simulink model "yamashev"  (R2015a)
settings: Solver=ode3  StartTime=0.0  StopTime=60.0  RelTol=1e-3
libraries: simulink x2, arduinolib x1
settings Model: ExtModeTrigDuration=2  Creator=maxim  LastModifiedBy=maxim
settings OptimizationCC: OptimizeModelRefInitCode=on  LifeSpan=1
settings DebuggingCC: UnderspecifiedInitializationDetection=Classic  MergeDetectMultiDrivingBlocksExec=none
settings HardwareCC: ProdBitPerInt=16  ProdBitPerPointer=8  ProdIntDivRoundTo=Zero  ProdEndianess=LittleEndian  ProdWordSize=8  ProdHWDeviceType=Atmel->AVR
settings RTWCC: SystemTargetFile=realtime.tlc  GenerateMakefile=off  TemplateMakefile=realtime.tmf  Description=Run on Target Hardware  RTWVerbose=off  CustomInclude=C:\Users\maxim\Documents\Arduino\libraries\OneWire C:\MATLAB\SupportPackages\R2015a\arduino-1.0.5\libraries\LiquidCrystal  CustomSource=C:\Users\maxim\Documents\Arduino\libraries\OneWire\OneWire.cpp C:\MATLAB\SupportPackages\R2015a\arduino-1.0.5\libraries\LiquidCrystal\LiquidCrystal.cpp DS18B20_03_custom.cpp LCD1602_02_custom.cpp
settings ERTTargetCC: CombineOutputUpdateFcns=off  ExtModeTransport=3  ExtModeMexFile=ext_serial_win32_comm_rtt  ExtModeMexArgs=0 1 9600  ERTSrcFileBannerTemplate=realtime_code_template.cgt  ERTHdrFileBannerTemplate=realtime_code_template.cgt  ERTDataSrcFileTemplate=realtime_code_template.cgt  ERTDataHdrFileTemplate=realtime_code_template.cgt  ERTCustomFileTemplate=realtime_file_process.tlc

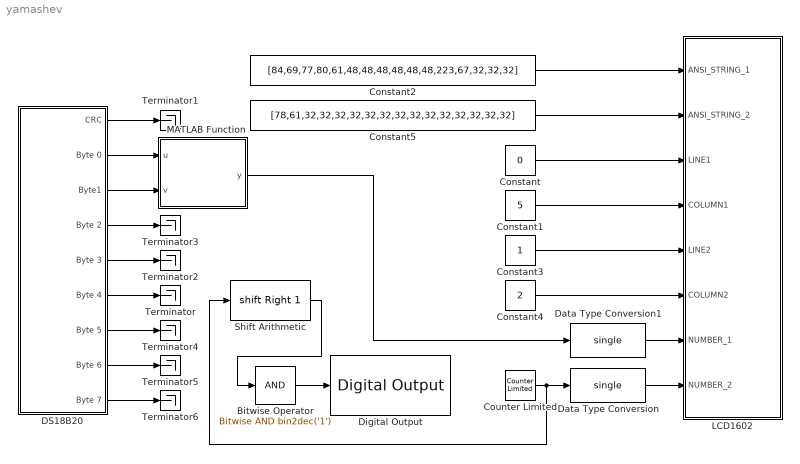
== system yamashev ==
  Bitwise Operator : simulink/Logic and Bit Operations/Bitwise Operator  logicop=AND  UseBitMask=on  BitMask=bin2dec('1')  BitMaskRealWorld=Stored Integer
  Constant : Constant  Value=0  OutDataTypeStr=uint8  LockScale=on
  Constant1 : Constant  Value=5  OutDataTypeStr=uint8  LockScale=on
  Constant2 : Constant  Value=[84,69,77,80,61,48,48,48,48,48,48,223,67,32,32,32]  OutDataTypeStr=fixdt('uint8', 'DataTypeOverride', 'Off')
  Constant3 : Constant  OutDataTypeStr=uint8
  Constant4 : Constant  Value=2  OutDataTypeStr=uint8  LockScale=on
  Constant5 : Constant  Value=[78,61,32,32,32,32,32,32,32,32,32,32,32,32,32,32]  OutDataTypeStr=uint8
  Counter Limited : simulink/Sources/Counter Limited  uplimit=100000  tsamp=-1
  DS18B20 : Subsystem  mask(DS18B20){PIN=34}
      mask prompts: PIN "PIN NUMBER"
      mask help:
      | Блок DS18B20 выполняет функции инициализации и считывания
      | измерений от цифрового термометра DS18B20, подключенного
      | по шине 1-Wire к отладочной плате Arduino Uno.
      | Параметры:
      | Pin Number: номер вывода отладочной платы Arduino Uno для
      | связи с DS18B20.
      | Выходные переменные:
      | CRC:8-разрядное значение контрольной суммы получаемое
      | от цифрового термометра DS18B20.
      | Byte0 ... Byte 7: байты пакета данных, передаваемые
      | от DS18B20.
      | Byte0: LSB младший 8-разрядный регистр температуры.
      | Byte1: MSB старший 8-разрядный регистр температуры.
      mask Help:
      | Блок DS18B20 выполняет функции инициализации и считывания измерений от
      | цифрового термометра DS18B20, подключенного по шине 1-Wire к порту
      | Pin Number отладочной платы Arduino Uno.
      | Параметры:
      | Pin Number: номер вывода Arduino Uno для связи с DS18B20.
      | Выходные переменные:
      | CRC: значение контрольной суммы получаемое от цифрового термометра DS18B20.
      | Byte0 ... Byte 7: байты пакета данных, передаваемые от DS18B20.
      | Byte0: LSB младший 8-разрядный регистр температуры.
      | Byte1: MSB старший 8-разрядный регистр температуры.
  Data Type Conversion : DataTypeConversion  OutDataTypeStr=single
  Data Type Conversion1 : DataTypeConversion  OutDataTypeStr=single
  Digital Output : arduinolib/Digital Output  pinNumber=32  blockPlatform=arduino
  LCD1602 : Subsystem  mask(LCD1602){RS=8, EN=9, D4=4, D5=5, D6=6, D7=7, CURSOR=0}
      mask prompts: RS "RS PIN"; EN "EN PIN"; D4 "D4 PIN"; D5 "D5 PIN"; D6 "D6 PIN"; D7 "D7 PIN"; CURSOR "CURSOR 1-ON 0-OFF"
      mask help:
      | Блок LCD1602 выполняет функции инициализации и вывода
      | информации на двухстрочный 16-символьный алфавитно-цифровой
      | ЖКИ-дисплей.Блок предназначен для работы на микроконтроллере
      | ATmega328 отладочной платы Arduino Uno в 4-битном режиме.
      | Параметры блока:
      | RS номер вывода Arduino Uno, подключаемый к контакту RS ЖКИ.
      | EN номер вывода Arduino Uno, подключаемый к контакту EN ЖКИ.
      | D4 номер вывода Arduino Uno, подключаемый к контакту D4 ЖКИ.
      | D5 номер вывода Arduino Uno, подключаемый к контакту D5 ЖКИ.
      | D6 номер вывода Arduino Uno, подключаемый к контакту D6 ЖКИ.
      | D7 номер вывода Arduino Uno, подключаемый к контакту D7 ЖКИ.
      | CURSOR: 1 – отображение курсора включено;
      |         0 – отображение курсора включено.
      | Входные переменные:
      | ANSI_STRING_1: 16-разрядный массив ANSI-кодов символов для вывода
      | на первую строку ЖКИ. (см. таблицу кодировок дисплея)
      | ANSI_STRING_1: 16-разрядный массив ANSI-кодов символов для вывода
      | на вторую строку ЖКИ. (см. таблицу кодировок дисплея)
      | LINE_1: 0/1 – номер строки для установки курсора вывода числа NUMBER_1.
      | COLUMN_1: 0, 1…15 – номер знакоместе в строке для установки курсора
      | вывода числа NUMBER_1.
      | LINE_2: 0/1 – номер строки для установки курсора вывода числа NUMBER_2.
      | COLUMN_2: 0, 1…15 – номер знакоместе в строке для установки курсора
      | вывода числа NUMBER_2.
      | NUMBER_1: первое числовое значение для отображения на дисплее.
      | NUMBER_2: второе числовое значение для отображения на дисплее.
      mask Help:
      | Блок LCD1602 выполняет функции инициализации и вывода информации на
      | двухстрочный 16-символьный алфавитно-цифровой ЖКИ-дисплей.
      | Блок предназначен для работы на микроконтроллере ATmega328 отладочной платы
      | Arduino Uno только в 4-битном режиме.
      | Параметры блока:
      | RS номер вывода Arduino Uno, подключаемый к контакту RS ЖКИ-модуля.
      | EN номер вывода Arduino Uno, подключаемый к контакту EN ЖКИ-модуля.
      | D4 номер вывода Arduino Uno, подключаемый к контакту D4 ЖКИ-модуля.
      | D5 номер вывода Arduino Uno, подключаемый к контакту D5 ЖКИ-модуля.
      | D6 номер вывода Arduino Uno, подключаемый к контакту D6 ЖКИ-модуля.
      | D7 номер вывода Arduino Uno, подключаемый к контакту D7 ЖКИ-модуля.
      | Входные переменные:
      | ANSI_STRING_1: 16-разрядный массив ANSI-кодов символов для вывода на первую
      | строку ЖКИ. (см. таблицу кодировок дисплея)
      | ANSI_STRING_1: 16-разрядный массив ANSI-кодов символов для вывода на вторую
      |  строку ЖКИ. (см. таблицу кодировок дисплея)
      | LINE_1: 0/1 – номер строки для установки курсора вывода числа NUMBER_1.
      | COLUMN_1: 0, 1…15 – номер знакоместе в строке для установки курсора
      | вывода числа NUMBER_1.
      | LINE_2: 0/1 – номер строки для установки курсора вывода числа NUMBER_2.
      | COLUMN_2: 0, 1…15 – номер знакоместе в строке для установки курсора
      | вывода числа NUMBER_2.
      | CursorSet: 1 – отображение курсора включено; 0 – отображение курсора включено.
      | NUMBER_1: первое числовое значение для отображения на дисплее.
      | NUMBER_2: второе числовое значение для отображения на дисплее.
      | Выходные переменные: отсутствуют.
  MATLAB Function : MATLAB Function  TreatAsAtomicUnit=on
  Shift Arithmetic : ArithShift  BitShiftNumber=1  BitShiftDirection=Right
  Terminator{,1..6} (7 alike) : Terminator
  wires:
  Constant/1 -> LCD1602/3(LINE1)
  Constant1/1 -> LCD1602/4(COLUMN1)
  Constant2/1 -> LCD1602/1(ANSI_STRING_1)
  DS18B20/8(Byte 6) -> Terminator5/1
  DS18B20/9(Byte 7) -> Terminator6/1
  DS18B20/7(Byte 5) -> Terminator4/1
  DS18B20/6(Byte 4) -> Terminator/1
  DS18B20/5(Byte 3) -> Terminator2/1
  DS18B20/4(Byte 2) -> Terminator3/1
  DS18B20/1(CRC) -> Terminator1/1
  Data Type Conversion/1 -> LCD1602/8(NUMBER_2)
  Constant3/1 -> LCD1602/5(LINE2)
  Constant4/1 -> LCD1602/6(COLUMN2)
  Constant5/1 -> LCD1602/2(ANSI_STRING_2)
  Data Type Conversion1/1 -> LCD1602/7(NUMBER_1)
  DS18B20/3(Byte1) -> MATLAB Function/2(v)
  MATLAB Function/1(y) -> Data Type Conversion1/1
  DS18B20/2(Byte 0) -> MATLAB Function/1(u)
  Counter Limited/1 -> Shift Arithmetic/1, Data Type Conversion/1
  Bitwise Operator/1 -> Digital Output/1
  Shift Arithmetic/1 -> Bitwise Operator/1

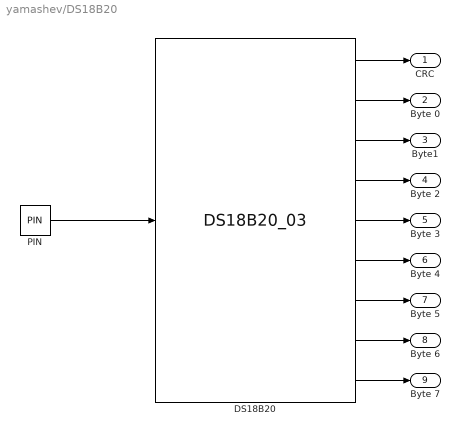
== system yamashev/DS18B20 ==
  DS18B20 : S-Function  InitFcn=try, set_param(gcb,'FunctionName','DS18B20_03'), end  FunctionName=DS18B20_03  SFunctionModules=DS18B20_03_wrapper  mask(S-Function Builder){}
      mask help: Simulink:masks:SFunctionBuilder_MD
      mask init:
      | val = [[.9  0.75 0.75 1 1 .9 .9 1]',[1 1 0.75 0.75 .9 .9 1 .9]'];try , sys = get_param(gcb,'SfunBuilderFcnName');if isempty(sys), sys = get_param(gcb,'FunctionName'); end,catch, sys = get_param(gcb,'FunctionName'); end
      settings: CopyFcn=set_param(gcbh,'LinkStatus','none')  PreSaveFcn=try, set_param(gcb,'FunctionName','DS18B20_03'), end  OpenFcn=sfunctionwizard(gcbh)
      mask Display: plot(val(:,1),val(:,2)),disp(sys), port_label('input',1,'PIN'), port_label('output',1,'CRC'), port_label('output',2,'BYTE0'), port_label('output',3,'BYTE1'), port_label('output',4,'BYTE2'), port_label('output',5,'BYTE3'), port_label('output',6,'BYTE4'), port_label('output',7,'BYTE5'), port_label('output',8,'BYTE6'), port_label('output',9,'BYTE7')
  PIN : Constant  Value=PIN  OutDataTypeStr=uint8
  CRC : Outport
  Byte 0 : Outport  Port=2
  Byte1 : Outport  Port=3
  Byte 2 : Outport  Port=4
  Byte 3 : Outport  Port=5
  Byte 4 : Outport  Port=6
  Byte 5 : Outport  Port=7
  Byte 6 : Outport  Port=8
  Byte 7 : Outport  Port=9
  wires:
  PIN/1 -> DS18B20/1
  DS18B20/9 -> Byte 7/1
  DS18B20/8 -> Byte 6/1
  DS18B20/7 -> Byte 5/1
  DS18B20/6 -> Byte 4/1
  DS18B20/5 -> Byte 3/1
  DS18B20/4 -> Byte 2/1
  DS18B20/3 -> Byte1/1
  DS18B20/2 -> Byte 0/1
  DS18B20/1 -> CRC/1

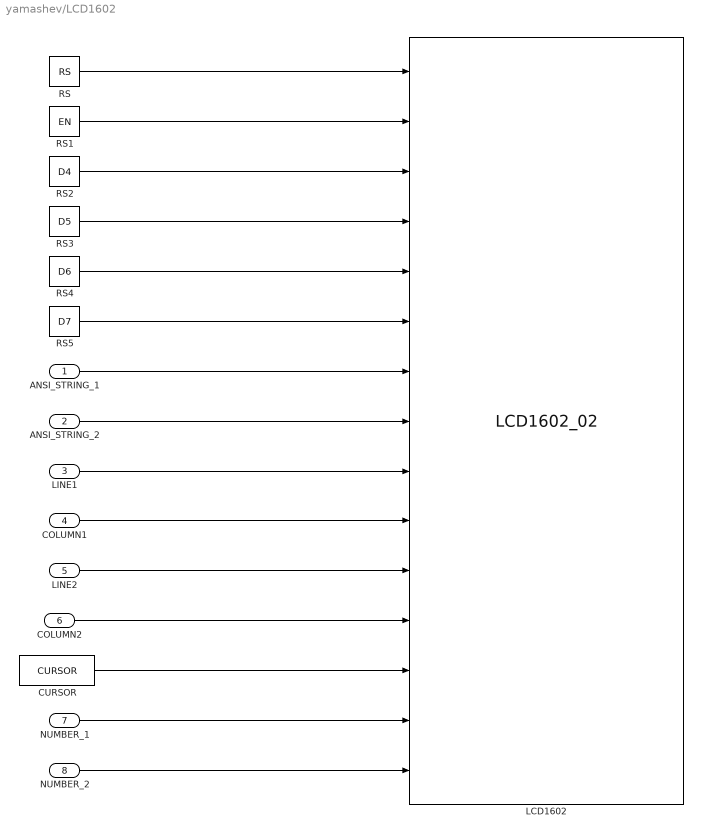
== system yamashev/LCD1602 ==
  ANSI_STRING_1 : Inport
  ANSI_STRING_2 : Inport  Port=2
  LINE1 : Inport  Port=3
  COLUMN1 : Inport  Port=4
  LINE2 : Inport  Port=5
  COLUMN2 : Inport  Port=6
  NUMBER_1 : Inport  Port=7
  NUMBER_2 : Inport  Port=8
  CURSOR : Constant  Value=CURSOR  OutDataTypeStr=uint8
  LCD1602 : S-Function  InitFcn=try, set_param(gcb,'FunctionName','LCD1602_02'), end  FunctionName=LCD1602_02  SFunctionModules=LCD1602_02_wrapper  mask(S-Function Builder){}
      mask help: Simulink:masks:SFunctionBuilder_MD
      mask init: same as yamashev/DS18B20/DS18B20
      settings: CopyFcn=set_param(gcbh,'LinkStatus','none')  PreSaveFcn=try, set_param(gcb,'FunctionName','LCD1602_02'), end  OpenFcn=sfunctionwizard(gcbh)
      mask Display: plot(val(:,1),val(:,2)),disp(sys), port_label('input',1,'RS_PIN'), port_label('input',2,'EN_PIN'), port_label('input',3,'D4_PIN'), port_label('input',4,'D5_PIN'), port_label('input',5,'D6_PIN'), port_label('input',6,'D7_PIN'), port_label('input',7,'SYMBOL_CODE_1'), port_label('input',8,'SYMBOL_CODE_2'), port_label('input',9,'LINE_1'), port_label('input',10,'COLUMN_1'), port_label('input',11,'LINE_2'), port_label('input',12,'COLUMN_2'), port_label('input',13,'CURSOR_ON'), port_label('input',14,'NUMBER_1'), port_label('input',15,'NUMBER_2')
  RS : Constant  Value=RS  OutDataTypeStr=uint8
  RS1 : Constant  Value=EN  OutDataTypeStr=uint8
  RS2 : Constant  Value=D4  OutDataTypeStr=uint8
  RS3 : Constant  Value=D5  OutDataTypeStr=uint8
  RS4 : Constant  Value=D6  OutDataTypeStr=uint8
  RS5 : Constant  Value=D7  OutDataTypeStr=uint8
  wires:
  LINE2/1 -> LCD1602/11
  COLUMN2/1 -> LCD1602/12
  CURSOR/1 -> LCD1602/13
  NUMBER_2/1 -> LCD1602/15
  NUMBER_1/1 -> LCD1602/14
  COLUMN1/1 -> LCD1602/10
  LINE1/1 -> LCD1602/9
  ANSI_STRING_2/1 -> LCD1602/8
  ANSI_STRING_1/1 -> LCD1602/7
  RS5/1 -> LCD1602/6
  RS4/1 -> LCD1602/5
  RS3/1 -> LCD1602/4
  RS2/1 -> LCD1602/3
  RS1/1 -> LCD1602/2
  RS/1 -> LCD1602/1

== matlab function yamashev/MATLAB Function ==
  data: u input; y output; v input
function y = combine(u, v)
    y = bitor(bitshift(v, 8), bitand(u, 255)) / 2.0;
end
